simulink model "proportional_controller"  (R2017a)
settings: Solver=VariableStepAuto  StartTime=0.0  StopTime=10.0  RelTol=1e-3
settings Model: Creator=adityaaaap  LastModifiedBy=adityaaaap

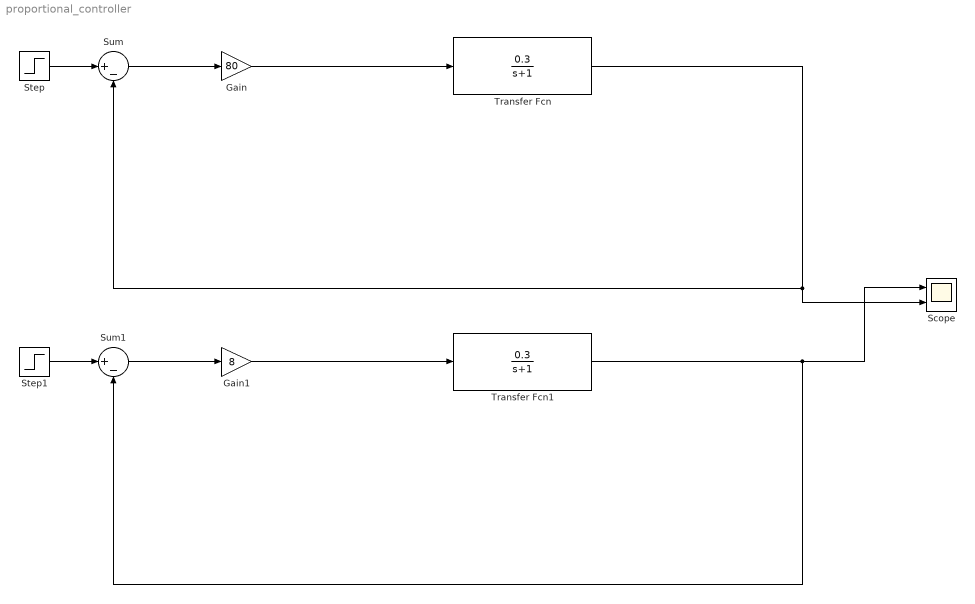
== system proportional_controller ==
  Gain : Gain  Gain=80
  Gain1 : Gain  Gain=8
  Scope : Scope  NumInputPorts=2
  Step : Step  Time=0  SampleTime=0
  Step1 : Step  Time=0  SampleTime=0
  Sum : Sum  Inputs=|+-
  Sum1 : Sum  Inputs=|+-
  Transfer Fcn : TransferFcn  Numerator=[0.3]  Denominator=[1 1]
  Transfer Fcn1 : TransferFcn  Numerator=[0.3]  Denominator=[1 1]
  wires:
  Sum/1 -> Gain/1
  Gain/1 -> Transfer Fcn/1
  Transfer Fcn/1 -> Sum/2, Scope/2
  Step/1 -> Sum/1
  Transfer Fcn1/1 -> Scope/1, Sum1/2
  Step1/1 -> Sum1/1
  Sum1/1 -> Gain1/1
  Gain1/1 -> Transfer Fcn1/1
